simulink model "steamjacket_test"  (R2019a)
settings: Solver=VariableStepAuto  StartTime=0.0  StopTime=100  RelTol=1e-3
settings Model: Creator=Adam  LastModifiedBy=Adam

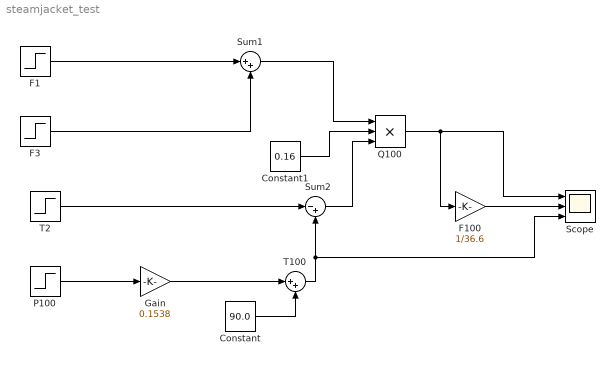
== system steamjacket_test ==
  Constant : Constant  Value=90.0
  Constant1 : Constant  Value=0.16
  F1 : Step  SampleTime=0
  F100 : Gain  Gain=1/36.6
  F3 : Step  SampleTime=0
  Gain : Gain  Gain=0.1538
  P100 : Step  SampleTime=0
  Q100 : Product  Inputs=3
  Scope : Scope  NumInputPorts=3
  Sum1 : Sum  Inputs=|++
  Sum2 : Sum  Inputs=|-+
  T100 : Sum  Inputs=|++
  T2 : Step  SampleTime=0
  wires:
  Constant/1 -> T100/2
  P100/1 -> Gain/1
  Gain/1 -> T100/1
  T100/1 -> Scope/3, Sum2/2
  F1/1 -> Sum1/1
  F3/1 -> Sum1/2
  T2/1 -> Sum2/1
  Sum1/1 -> Q100/1
  Constant1/1 -> Q100/2
  Sum2/1 -> Q100/3
  Q100/1 -> Scope/1, F100/1
  F100/1 -> Scope/2
